simulink model "Linearizzazione_fellata_lqi"  (R2025b)
settings: Solver=VariableStepAuto  StartTime=0.0  StopTime=10.0  RelTol=1e-3
undefined symbols (not defined in the file): A, B, K_lqi, nu, nx, x0
settings Model: Creator=Miche  LastModifiedBy=Miche

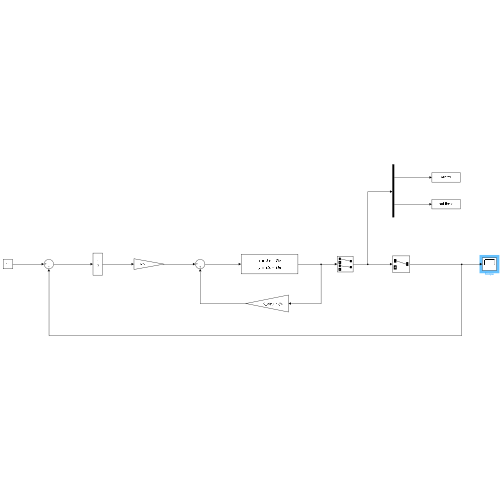
[thumbnail: Simulink's stored preview of the top-level diagram]
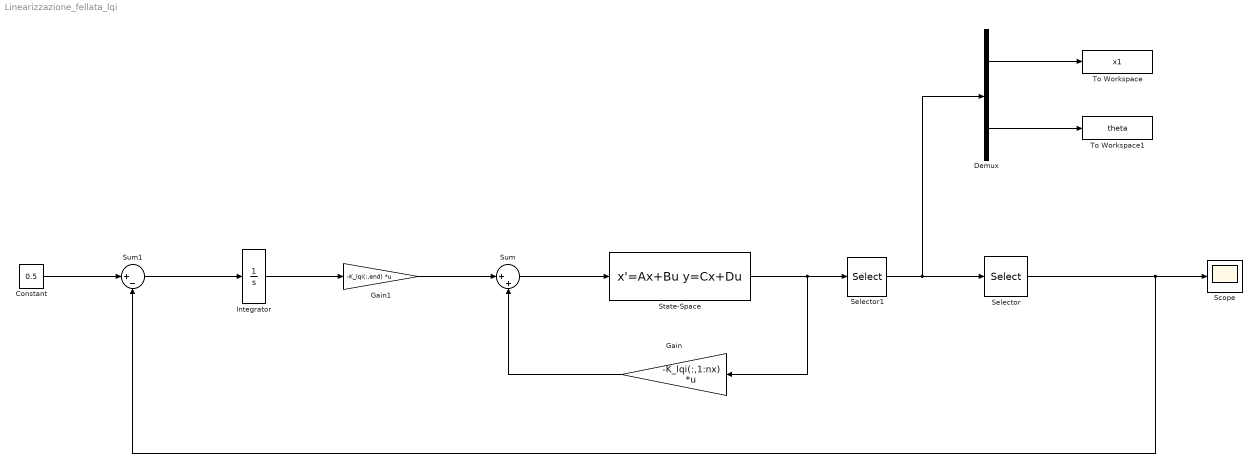
== system Linearizzazione_fellata_lqi ==
  Constant : Constant  Value=0.5
  Demux : Demux  Outputs=2
  Gain : Gain  Gain=-K_lqi(:,1:nx)  Multiplication=Matrix(K*u)
  Gain1 : Gain  Gain=-K_lqi(:,end)  Multiplication=Matrix(K*u)
  Integrator : Integrator
  Scope : Scope
      settings: ActiveDisplayYMinimum=0.036424076678425982  ActiveDisplayYMaximum=0.5515395285481981
  Selector : Selector  InputPortWidth=2  IndexOptions=Index vector (dialog)  Indices=1  OutputSizes=1
  Selector1 : Selector  InputPortWidth=4  IndexOptions=Index vector (dialog)  Indices=[1 3]  OutputSizes=1
  State-Space : StateSpace  A=A  B=B  C=eye(nx)  D=zeros(nx,nu)  InitialCondition=x0
  Sum : Sum  Inputs=|++
  Sum1 : Sum  Inputs=|+-
  To Workspace : ToWorkspace  VariableName=x1  SaveFormat=Timeseries  SampleTime=-1
  To Workspace1 : ToWorkspace  VariableName=theta  SaveFormat=Timeseries  SampleTime=-1
  wires:
  Gain/1 -> Sum/2
  Sum/1 -> State-Space/1
  Integrator/1 -> Gain1/1
  Gain1/1 -> Sum/1
  State-Space/1 -> Selector1/1, Gain/1
  Sum1/1 -> Integrator/1
  Demux/1 -> To Workspace/1
  Selector/1 -> Sum1/2, Scope/1
  Demux/2 -> To Workspace1/1
  Constant/1 -> Sum1/1
  Selector1/1 -> Demux/1, Selector/1
